simulink model "MCModel"  (R2020b)
settings: Solver=VariableStepAuto  StartTime=0.0  StopTime=4  RelTol=1e-3
libraries: mcbcontrolslib x7, mcbpositiondecoderlib x1, autolibpmsmexterior x1
settings Model: Creator=leoja  LastModifiedBy=leoja

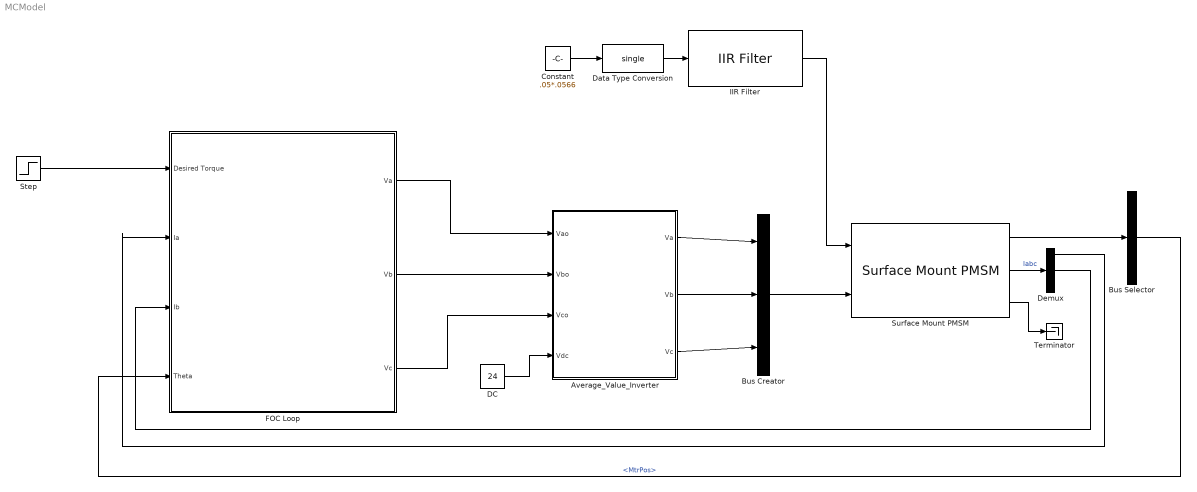
== system MCModel ==
  Average_Value_Inverter : Subsystem
  Bus Creator : BusCreator  Inputs=3
  Bus Selector : BusSelector  OutputSignals=MtrPos
  Constant : Constant  Value=.05*.0566
  "DC " : Constant  Value=24
  Data Type Conversion : DataTypeConversion  OutDataTypeStr=single
  Demux : Demux  Outputs=3
  FOC Loop : Subsystem
  IIR Filter : mcbcontrolslib/IIR Filter  Filter_constant=0.01
      settings: SourceProductBaseCode=MT
  Step : Step  Time=2  SampleTime=0
  Surface Mount PMSM : autolibpmsmexterior/Surface Mount PMSM  port_config=Torque  sim_type=Discrete  Ts=2.5e-5  FilePath=E:\Sandbox\Bauto\Work\surfacepmsm_motordata.m  P=4  Rs=.75  Ldq_=.0011  KConstText=Permanent flux linkage constant (lambda_pm):  lambda_pm=.0052  Ke=159.9771  Kt=1.323  mechanical=[2.4e-6, 1.16e-5, 0]  idq0=[0 0]  theta_init=0  omega_init=0  KConst=.0052  lambda_pm_calc=.0052  RefBlkName='autolibpmsmexterior/Surface Mount PMSM'  aMode=5  Ldq="[0.00105     0.00105]"
      settings: SourceProductBaseCode=PW,MT,UV,VE,VP
  Terminator : Terminator
  wires:
  FOC Loop/1(Va) -> Average_Value_Inverter/1(Vao)
  FOC Loop/2(Vb) -> Average_Value_Inverter/2(Vbo)
  FOC Loop/3(Vc) -> Average_Value_Inverter/3(Vco)
  Average_Value_Inverter/1(Va) -> Bus Creator/1
  Average_Value_Inverter/2(Vb) -> Bus Creator/2
  Average_Value_Inverter/3(Vc) -> Bus Creator/3
  Bus Creator/1 -> Surface Mount PMSM/2
  Surface Mount PMSM/1 -> Bus Selector/1
  Bus Selector/1 -> FOC Loop/4(Theta)  "<MtrPos>"
  Surface Mount PMSM/2 -> Demux/1  "Iabc"
  Demux/1 -> FOC Loop/2(Ia)
  Demux/2 -> FOC Loop/3(Ib)
  Step/1 -> FOC Loop/1(Desired Torque)
  "DC "/1 -> Average_Value_Inverter/4(Vdc)
  Constant/1 -> Data Type Conversion/1
  Data Type Conversion/1 -> IIR Filter/1
  IIR Filter/1 -> Surface Mount PMSM/1
  Surface Mount PMSM/3 -> Terminator/1

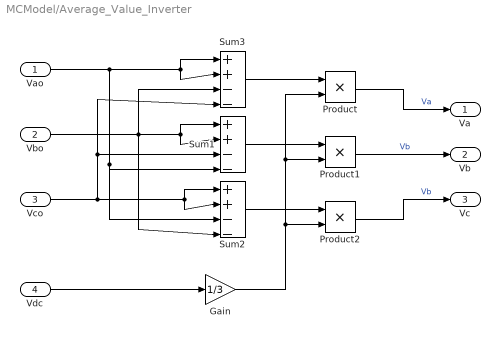
== system MCModel/Average_Value_Inverter ==
  Vao : Inport
  Vbo : Inport  Port=2
  Vco : Inport  Port=3
  Vdc : Inport  Port=4
  Gain : Gain  Gain=1/3  RndMeth=Simplest  OutDataTypeStr=Inherit: Same as input
  Product : Product  RndMeth=Simplest  OutDataTypeStr=Inherit: Same as first input
  Product1 : Product  RndMeth=Simplest  OutDataTypeStr=Inherit: Same as first input
  Product2 : Product  RndMeth=Simplest  OutDataTypeStr=Inherit: Same as first input
  Sum1 : Sum  Inputs=|++--  RndMeth=Simplest  OutDataTypeStr=Inherit: Same as first input
  Sum2 : Sum  Inputs=|++--  RndMeth=Simplest  OutDataTypeStr=Inherit: Same as first input
  Sum3 : Sum  Inputs=|++--  RndMeth=Simplest  OutDataTypeStr=Inherit: Same as first input
  Va : Outport  VectorParamsAs1DForOutWhenUnconnected=off
  Vb : Outport  Port=2  VectorParamsAs1DForOutWhenUnconnected=off
  Vc : Outport  Port=3  VectorParamsAs1DForOutWhenUnconnected=off
  wires:
  Product1/1 -> Vb/1  "Vb"
  Gain/1 -> Product/2, Product1/2, Product2/2
  Sum2/1 -> Product2/1
  Vao/1 -> Sum3/1, Sum3/2, Sum1/4, Sum2/3
  Product2/1 -> Vc/1  "Vb"
  Sum1/1 -> Product1/1
  Vdc/1 -> Gain/1
  Sum3/1 -> Product/1
  Product/1 -> Va/1  "Va"
  Vco/1 -> Sum3/4, Sum1/3, Sum2/2, Sum2/1
  Vbo/1 -> Sum1/1, Sum1/2, Sum3/3, Sum2/4

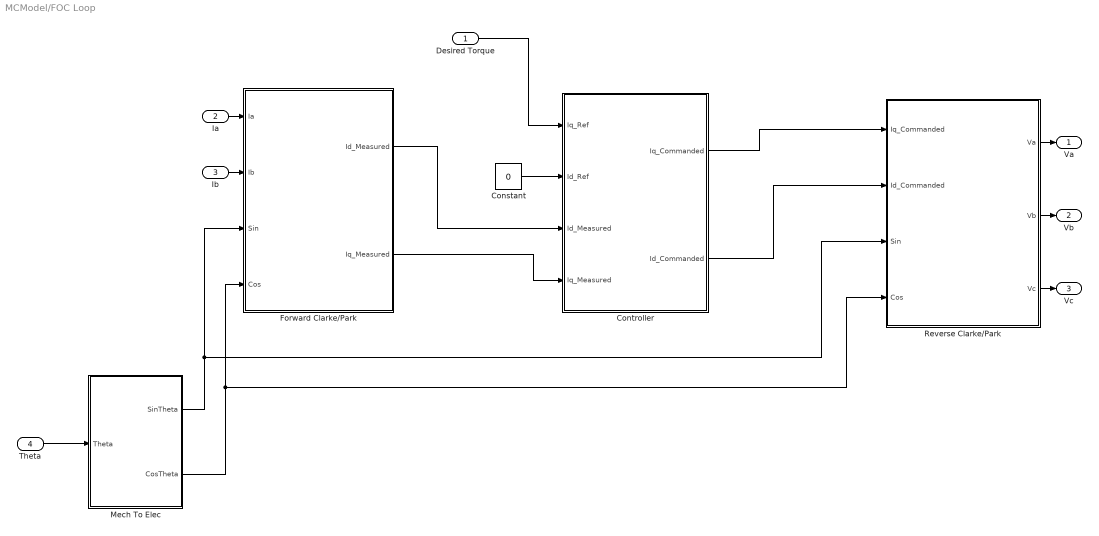
== system MCModel/FOC Loop ==
  Desired Torque : Inport
  Ia : Inport  Port=2
  Ib : Inport  Port=3
  Theta : Inport  Port=4
  Constant : Constant  Value=0
  Controller : Subsystem
  Forward Clarke/Park : Subsystem
  Mech To Elec : Subsystem
  Reverse Clarke/Park : Subsystem
  Va : Outport
  Vb : Outport  Port=2
  Vc : Outport  Port=3
  wires:
  Mech To Elec/1(SinTheta) -> Reverse Clarke/Park/3(Sin), Forward Clarke/Park/3(Sin)
  Mech To Elec/2(CosTheta) -> Forward Clarke/Park/4(Cos), Reverse Clarke/Park/4(Cos)
  Constant/1 -> Controller/2(Id_Ref)
  Controller/1(Iq_Commanded) -> Reverse Clarke/Park/1(Iq_Commanded)
  Controller/2(Id_Commanded) -> Reverse Clarke/Park/2(Id_Commanded)
  Forward Clarke/Park/2(Iq_Measured) -> Controller/4(Iq_Measured)
  Reverse Clarke/Park/3(Vc) -> Vc/1
  Forward Clarke/Park/1(Id_Measured) -> Controller/3(Id_Measured)
  Reverse Clarke/Park/1(Va) -> Va/1
  Reverse Clarke/Park/2(Vb) -> Vb/1
  Theta/1 -> Mech To Elec/1(Theta)
  Ib/1 -> Forward Clarke/Park/2(Ib)
  Ia/1 -> Forward Clarke/Park/1(Ia)
  Desired Torque/1 -> Controller/1(Iq_Ref)

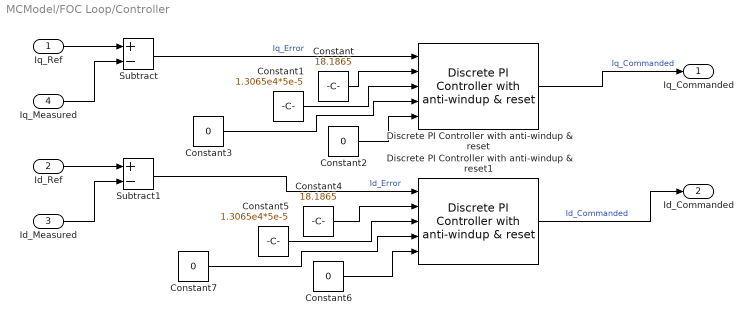
== system MCModel/FOC Loop/Controller ==
  Iq_Ref : Inport
  Id_Ref : Inport  Port=2
  Id_Measured : Inport  Port=3
  Iq_Measured : Inport  Port=4
  Constant : Constant  Value=18.1865
  Constant1 : Constant  Value=1.3065e4*5e-5
  Constant{2..3,6..7} (4 alike) : Constant  Value=0
  Constant4 : Constant  Value=18.1865
  Constant5 : Constant  Value=1.3065e4*5e-5
  Discrete PI Controller with anti-windup & reset : mcbcontrolslib/Discrete PI Controller  with anti-windup & reset  UpperSaturationLimit=1  LowerSaturationLimit=-1
      settings: SourceProductBaseCode=MT
  Discrete PI Controller with anti-windup & reset1 : mcbcontrolslib/Discrete PI Controller  with anti-windup & reset  UpperSaturationLimit=1  LowerSaturationLimit=-1
      settings: SourceProductBaseCode=MT
  Subtract : Sum  Inputs=+-
  Subtract1 : Sum  Inputs=+-
  Iq_Commanded : Outport
  Id_Commanded : Outport  Port=2
  wires:
  Subtract1/1 -> Discrete PI Controller with anti-windup & reset1/1  "Id_Error"
  Discrete PI Controller with anti-windup & reset1/1 -> Id_Commanded/1  "Id_Commanded"
  Subtract/1 -> Discrete PI Controller with anti-windup & reset/1  "Iq_Error"
  Iq_Measured/1 -> Subtract/2
  Discrete PI Controller with anti-windup & reset/1 -> Iq_Commanded/1  "Iq_Commanded"
  Id_Ref/1 -> Subtract1/1
  Iq_Ref/1 -> Subtract/1
  Id_Measured/1 -> Subtract1/2
  Constant/1 -> Discrete PI Controller with anti-windup & reset/2
  Constant1/1 -> Discrete PI Controller with anti-windup & reset/3
  Constant2/1 -> Discrete PI Controller with anti-windup & reset/5
  Constant3/1 -> Discrete PI Controller with anti-windup & reset/4
  Constant6/1 -> Discrete PI Controller with anti-windup & reset1/5
  Constant7/1 -> Discrete PI Controller with anti-windup & reset1/4
  Constant4/1 -> Discrete PI Controller with anti-windup & reset1/2
  Constant5/1 -> Discrete PI Controller with anti-windup & reset1/3

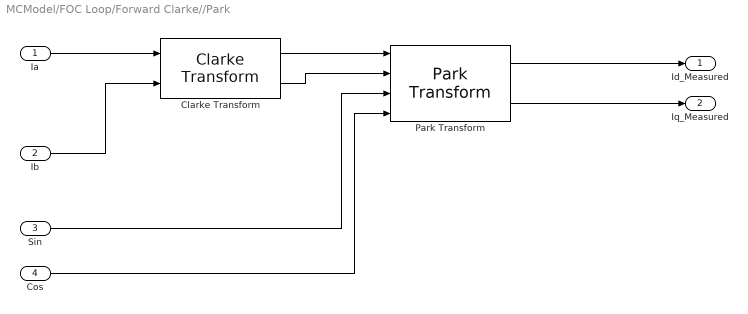
== system MCModel/FOC Loop/Forward Clarke//Park ==
  Ia : Inport
  Ib : Inport  Port=2
  Sin : Inport  Port=3
  Cos : Inport  Port=4
  Clarke Transform : mcbcontrolslib/Clarke Transform  VariantControl=Variant2
  Park Transform : mcbcontrolslib/Park Transform  AxisAlignment=D-axis
      settings: SourceProductBaseCode=MT
  Id_Measured : Outport
  Iq_Measured : Outport  Port=2
  wires:
  Ia/1 -> Clarke Transform/1
  Ib/1 -> Clarke Transform/2
  Clarke Transform/1 -> Park Transform/1
  Clarke Transform/2 -> Park Transform/2
  Sin/1 -> Park Transform/3
  Cos/1 -> Park Transform/4
  Park Transform/1 -> Id_Measured/1
  Park Transform/2 -> Iq_Measured/1

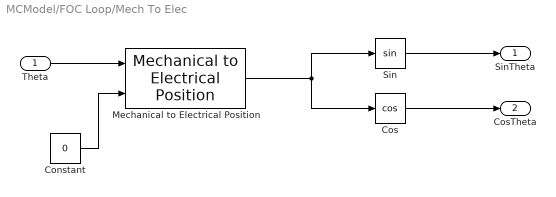
== system MCModel/FOC Loop/Mech To Elec ==
  Theta : Inport
  Constant : Constant  Value=0
  Cos : Trigonometry  Operator=cos
  Mechanical to Electrical Position : mcbpositiondecoderlib/Mechanical to Electrical Position  NrPP=6  selectedRange=Per unit  MechOfstInputType=Input port  mechOffsetIn=0  maxAngleIn=1  InputDataType=single  VariantSelect=floating-point
      settings: SourceProductBaseCode=MT
  Sin : Trigonometry
  SinTheta : Outport
  CosTheta : Outport  Port=2
  wires:
  Mechanical to Electrical Position/1 -> Cos/1, Sin/1
  Constant/1 -> Mechanical to Electrical Position/2
  Theta/1 -> Mechanical to Electrical Position/1
  Sin/1 -> SinTheta/1
  Cos/1 -> CosTheta/1

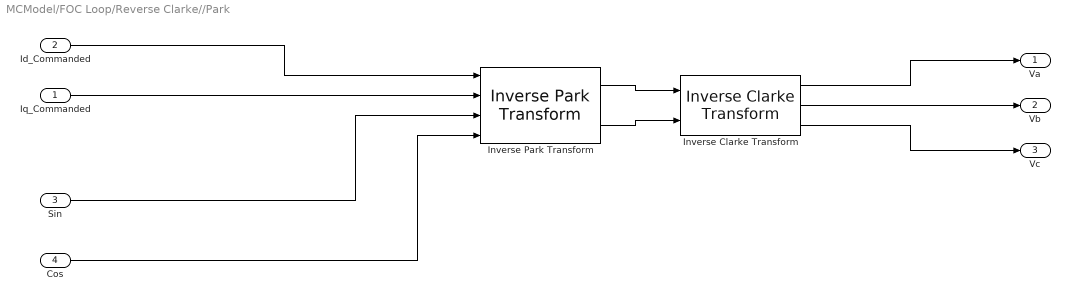
== system MCModel/FOC Loop/Reverse Clarke//Park ==
  Iq_Commanded : Inport
  Id_Commanded : Inport  Port=2
  Sin : Inport  Port=3
  Cos : Inport  Port=4
  Inverse Clarke Transform : mcbcontrolslib/Inverse Clarke Transform
      settings: SourceProductBaseCode=MT
  Inverse Park Transform : mcbcontrolslib/Inverse Park Transform  AxisAlignment=D-axis
  Va : Outport
  Vb : Outport  Port=2
  Vc : Outport  Port=3
  wires:
  Inverse Park Transform/1 -> Inverse Clarke Transform/1
  Inverse Park Transform/2 -> Inverse Clarke Transform/2
  Inverse Clarke Transform/1 -> Va/1
  Inverse Clarke Transform/2 -> Vb/1
  Inverse Clarke Transform/3 -> Vc/1
  Sin/1 -> Inverse Park Transform/3
  Cos/1 -> Inverse Park Transform/4
  Id_Commanded/1 -> Inverse Park Transform/1
  Iq_Commanded/1 -> Inverse Park Transform/2
